simulink model "gm_BER_calc"  (R2016b)
settings: Solver=VariableStepAuto  StartTime=0.0  StopTime=256  RelTol=1e-3
undefined symbols (not defined in the file or in its folder): det_data, true_data
libraries: hdlsllib x3
settings Model: Creator=Arthur  LastModifiedBy=Arthur
settings OptimizationCC: DefaultParameterBehavior=Inlined
settings DebuggingCC: StrictBusMsg=ErrorOnBusTreatedAsVector

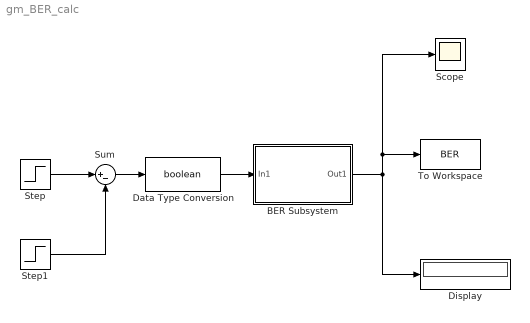
== system gm_BER_calc ==
  BER Subsystem : Subsystem
  Data Type Conversion : DataTypeConversion  OutDataTypeStr=boolean
  Display : Display
  Scope : Scope
  Step : Step  Time=0  SampleTime=1
  Step1 : Step  SampleTime=1
  Sum : Sum  Inputs=|+-
  To Workspace : ToWorkspace  VariableName=BER  SampleTime=-1
  wires:
  Step1/1 -> Sum/2
  Step/1 -> Sum/1
  Sum/1 -> Data Type Conversion/1
  BER Subsystem/1(Out1) -> Scope/1, To Workspace/1, Display/1
  Data Type Conversion/1 -> BER Subsystem/1(In1)

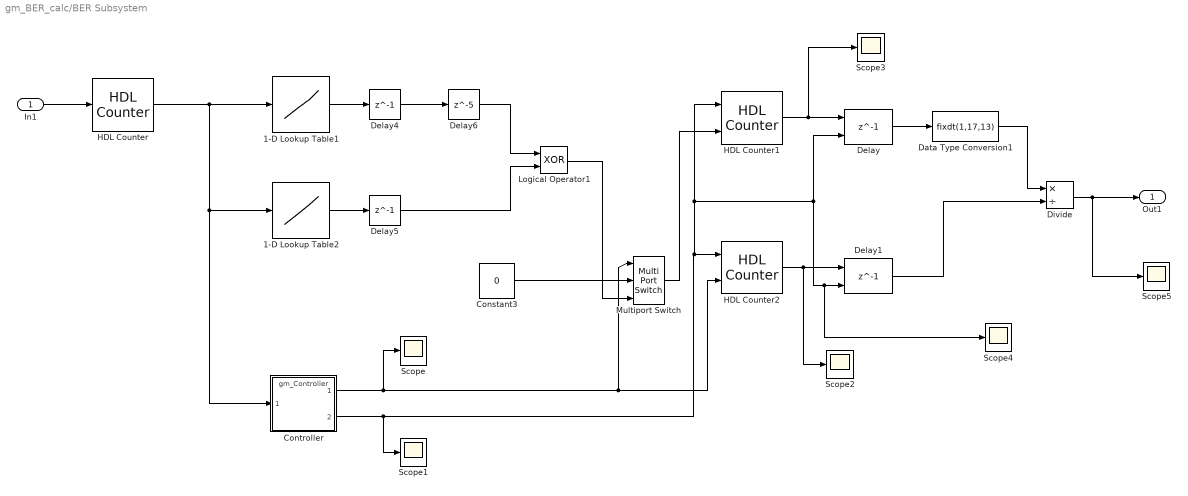
== system gm_BER_calc/BER Subsystem ==
  In1 : Inport
  1-D Lookup Table1 : Lookup_n-D  NumberOfTableDimensions=1  BreakpointsForDimension1=[0:255]  BreakpointsForDimension1FirstPoint=10  BreakpointsForDimension2FirstPoint=10  BreakpointsForDimension1Spacing=12  BreakpointsForDimension2Spacing=12  IndexSearchMethod=Evenly spaced points  Table=true_data*1  InterpMethod=Flat  DiagnosticForOutOfRangeInput=Error  InternalRulePriority=Speed  RndMeth=Simplest  InputSameDT=on
  1-D Lookup Table2 : Lookup_n-D  NumberOfTableDimensions=1  BreakpointsForDimension1=[0:255]  BreakpointsForDimension1FirstPoint=10  BreakpointsForDimension2FirstPoint=10  BreakpointsForDimension1Spacing=12  BreakpointsForDimension2Spacing=12  IndexSearchMethod=Evenly spaced points  Table=det_data*1  InterpMethod=Flat  DiagnosticForOutOfRangeInput=Error  InternalRulePriority=Speed  RndMeth=Simplest  InputSameDT=on
  Constant3 : Constant  Value=0  VectorParams1D=off  OutDataTypeStr=boolean  SampleTime=-1
  Controller : ModelReference  ModelNameDialog=gm_Controller  SimulationMode=Normal  Variant=on  OverrideUsingVariant=HDLC_internal_variant_GeneratedDUT  ModelReferenceVersion=1.7
  Data Type Conversion1 : DataTypeConversion  OutDataTypeStr=fixdt(1,17,13)
  Delay : Delay  DelayLength=1  InitialCondition=0  ExternalReset=Rising  UseCircularBuffer=on
      settings: InputPortMap=u0,r5
  Delay1 : Delay  DelayLength=1  InitialCondition=0  ExternalReset=Rising  UseCircularBuffer=on
      settings: InputPortMap=u0,r5
  Delay4 : Delay  DelayLength=1
  Delay5 : Delay  DelayLength=1
  Delay6 : Delay  DelayLength=5
  Divide : Product  Inputs=*/  OutDataTypeStr=fixdt(1,17,13)
  HDL Counter : hdlsllib/HDL Operations/HDL Counter  CountType=Count limited  CountInit=0  CountStep=1  CountMax=255  CountFromType=Initial value  CountFrom=0  CountResetPort=on  CountLoadPort=off  CountEnbPort=off  CountDirPort=off  CountDataType=Signed  CountWordLen=17  CountFracLen=0  CountSampTime=1
  HDL Counter1 : hdlsllib/HDL Operations/HDL Counter  CountType=Free running  CountInit=0  CountStep=1  CountMax=25  CountFromType=Specify  CountFrom=0  CountResetPort=on  CountLoadPort=off  CountEnbPort=on  CountDirPort=off  CountDataType=Signed  CountWordLen=17  CountFracLen=0  CountSampTime=1
  HDL Counter2 : hdlsllib/HDL Operations/HDL Counter  CountType=Free running  CountInit=0  CountStep=1  CountMax=25  CountFromType=Specify  CountFrom=0  CountResetPort=on  CountLoadPort=off  CountEnbPort=on  CountDirPort=off  CountDataType=Signed  CountWordLen=17  CountFracLen=0  CountSampTime=1
  Logical Operator1 : Logic  Operator=XOR  AllPortsSameDT=off  OutDataTypeStr=boolean
  Multiport Switch : MultiPortSwitch  DataPortOrder=Zero-based contiguous  Inputs=2
  Scope{,1..5} (6 alike) : Scope
  Out1 : Outport
  wires:
  Delay4/1 -> Delay6/1
  Delay6/1 -> Logical Operator1/1
  Delay5/1 -> Logical Operator1/2
  Logical Operator1/1 -> Multiport Switch/3
  Controller/1 -> Scope/1, HDL Counter2/2, Multiport Switch/1
  Constant3/1 -> Multiport Switch/2
  Divide/1 -> Scope5/1, Out1/1
  HDL Counter2/1 -> Scope2/1, Delay1/1
  HDL Counter1/1 -> Scope3/1, Delay/1
  Delay1/1 -> Divide/2
  Data Type Conversion1/1 -> Divide/1
  Delay/1 -> Data Type Conversion1/1
  HDL Counter/1 -> 1-D Lookup Table1/1, 1-D Lookup Table2/1, Controller/1
  Controller/2 -> Scope1/1, Scope4/1, Delay1/2, Delay/2, HDL Counter1/1, HDL Counter2/1
  Multiport Switch/1 -> HDL Counter1/2
  In1/1 -> HDL Counter/1
  1-D Lookup Table2/1 -> Delay5/1
  1-D Lookup Table1/1 -> Delay4/1
